simulink model "Capstone_Model"  (R2022b)
settings: Solver=VariableStepAuto  StartTime=0.0  StopTime=10.0  RelTol=1e-3
libraries: sh_lib x6, fl_lib x5, nesl_utility x2, simulink x1
settings Model: Creator=jrodd  LastModifiedBy=jrodd

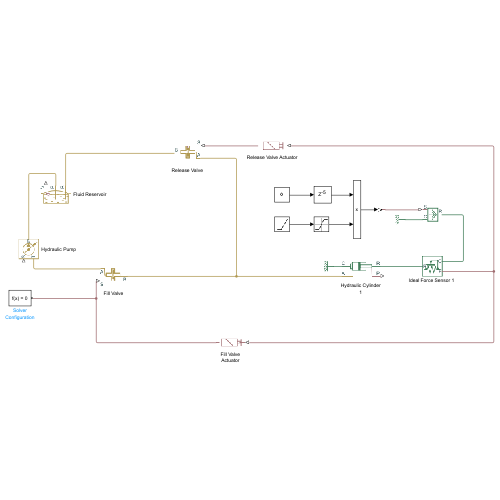
[thumbnail: Simulink's stored preview of the top-level diagram]
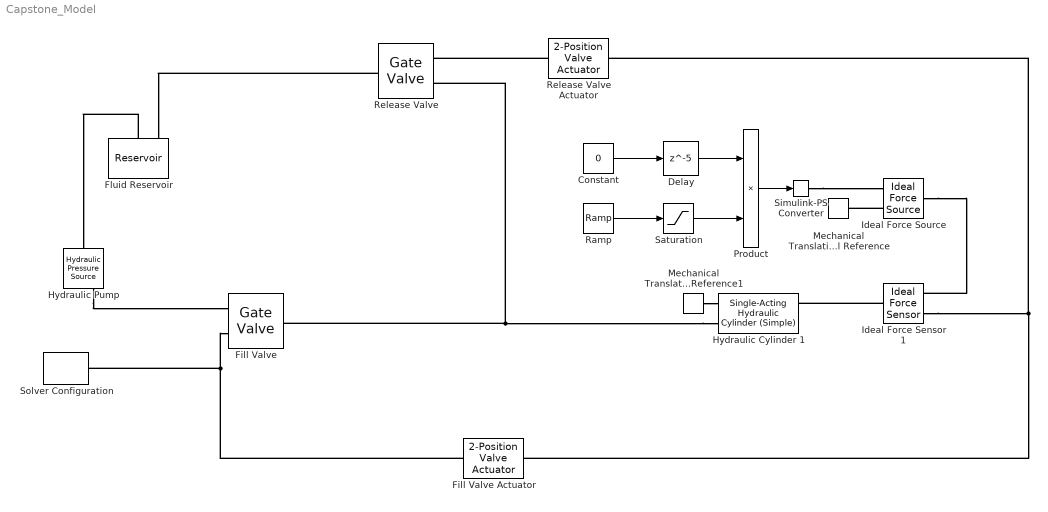
== system Capstone_Model ==
  Constant : Constant  Value=0
  Delay : Delay  DelayLength=5
  Fill Valve : sh_lib/Valves/Flow Control Valves/Gate Valve  d_gate=0.01 m  x_0=0 m  C_d=0.65  A_leak=1e-12 m^2  lam_spec=1  B_lam=0.999  Re_cr=10
      settings: InternalSimscapePortConfiguration="{\"Bottom\":[],\"Left\":[{\"id\":\"S\",\"label\":\"S\",\"type\":\"input\"},{\"id\":\"A\",\"label\":\"A\",\"type\":\"foundation.hydraulic.hydraulic\"}],\"Right\":[{\"id\":\"B\",\"label\":\"B\",\"type\":\"foundation.hydraulic.hydraulic\"}],\"Top\":[]}"
  Fill Valve Actuator : sh_lib/Valves/Valve Actuators/2-Position Valve Actuator  stroke=0.01 m  t_on=0.1 s  t_off=0.1 s  act_signal=1  init_position=0  act_orientation=1
      settings: InternalSimscapePortConfiguration="{\"Bottom\":[],\"Left\":[{\"id\":\"C\",\"label\":\"\",\"type\":\"input\"}],\"Right\":[{\"id\":\"P\",\"label\":\"\",\"type\":\"output\"}],\"Top\":[]}"
  Fluid Reservoir : sh_lib/Hydraulic Utilities/Reservoir  press=0 Pa  init_volume=0.02 m^3  ret_diam=0.02 m  loss_coeff=1
      settings: InternalSimscapePortConfiguration="{\"Bottom\":[],\"Left\":[{\"id\":\"V\",\"label\":\"V\",\"type\":\"output\"},{\"id\":\"P\",\"label\":\"P\",\"type\":\"foundation.hydraulic.hydraulic\"},{\"id\":\"R\",\"label\":\"R\",\"type\":\"foundation.hydraulic.hydraulic\"}],\"Right\":[],\"Top\":[]}"
  Hydraulic Cylinder 1 : sh_lib/Hydraulic Cylinders/Single-Acting Hydraulic Cylinder (Simple)  area=5e-4 m^2  stroke=0.1 m  init_pos=0 m  penetr_coeff=1e12 N*s/m^2  or=1
      settings: InternalSimscapePortConfiguration="{\"Bottom\":[],\"Left\":[{\"id\":\"C\",\"label\":\"C\",\"type\":\"foundation.mechanical.translational.translational\"},{\"id\":\"A\",\"label\":\"A\",\"type\":\"foundation.hydraulic.hydraulic\"}],\"Right\":[{\"id\":\"R\",\"label\":\"R\",\"type\":\"foundation.mechanical.translational.translational\"},{\"id\":\"P\",\"label\":\"P\",\"type\":\"output\"}],\"Top\":[]}"
  Hydraulic Pump : fl_lib/Hydraulic/Hydraulic Sources/Hydraulic Pressure Source
      settings: InternalSimscapePortConfiguration="{\"Bottom\":[],\"Left\":[{\"id\":\"P\",\"label\":\"P\",\"type\":\"foundation.hydraulic.hydraulic\"}],\"Right\":[{\"id\":\"S\",\"label\":\"S\",\"type\":\"input\"},{\"id\":\"T\",\"label\":\"T\",\"type\":\"foundation.hydraulic.hydraulic\"}],\"Top\":[]}"
  "Ideal Force Sensor 1 " : fl_lib/Mechanical/Mechanical Sensors/Ideal Force Sensor
  Ideal Force Source : fl_lib/Mechanical/Mechanical Sources/Ideal Force Source
  Mechanical Translational Reference : fl_lib/Mechanical/Translational Elements/Mechanical Translational Reference
  Mechanical Translational Reference1 : fl_lib/Mechanical/Translational Elements/Mechanical Translational Reference
  Product : Product
  Ramp : simulink/Sources/Ramp  slope=1  start=1  InitialOutput=0
  Release Valve : sh_lib/Valves/Flow Control Valves/Gate Valve  d_gate=0.01 m  x_0=0 m  C_d=0.65  A_leak=1e-12 m^2  lam_spec=1  B_lam=0.999  Re_cr=10
      settings: InternalSimscapePortConfiguration="{\"Bottom\":[],\"Left\":[{\"id\":\"S\",\"label\":\"S\",\"type\":\"input\"},{\"id\":\"A\",\"label\":\"A\",\"type\":\"foundation.hydraulic.hydraulic\"}],\"Right\":[{\"id\":\"B\",\"label\":\"B\",\"type\":\"foundation.hydraulic.hydraulic\"}],\"Top\":[]}"
  Release Valve Actuator : sh_lib/Valves/Valve Actuators/2-Position Valve Actuator  stroke=0.01 m  t_on=0.1 s  t_off=0.1 s  act_signal=1  init_position=1  act_orientation=1
      settings: InternalSimscapePortConfiguration="{\"Bottom\":[],\"Left\":[{\"id\":\"C\",\"label\":\"\",\"type\":\"input\"}],\"Right\":[{\"id\":\"P\",\"label\":\"\",\"type\":\"output\"}],\"Top\":[]}"
  Saturation : Saturate  UpperLimit=2  LowerLimit=0
  Simulink-PS Converter : nesl_utility/Simulink-PS Converter  PhysicalDomain=network_engine_domain  SubClassName=ps_input  LeftPortType=input  RightPortType=output  PseudoPeriodic=off  Frequencies=[]  NoiseDistribution=none  NoiseParameters=[]  Unit=1  AffineConversion=off  FilteringAndDerivatives=provide  SimscapeFilterOrder=1  InputFilterTimeConstant=0.001  UdotUserProvided=0
  Solver Configuration : nesl_utility/Solver Configuration  PhysicalDomain=network_engine_domain  SubClassName=solver  LeftPortType=input  RightPortType=generic  Tones=[]  Harmonics=[]  SimulateNoise=off  Profile=off  UseLocalSampling=off  EnableSwitchedLinearOptims=on  FrequencyDomain=off  UseCCode=off  RelTol=0.001  AbsTol=0.001  MinStep=1e-09  ToWorkspace=off  RevertToSquareIcSolve=off  NumHomotopyIterations=100  PhasorMode=off  PhasorModeNumHarmonics=1  ConsistencySolver=NEWTON_XTOL_AFTER_FTOL  IndexReductionMethod=DerivativeReplacement  DoDC=off  ResidualTolerance=1e-09  ConsistencyTolSource=GLOBAL  ConsistencyAbsTol=0.001  ConsistencyRelTol=0.001  ConsistencyTolFactor=0.001  UseLocalSolver=off  LocalSolverChoice=NE_BACKWARD_EULER_ADVANCER  ResolveIndetEquations=on  FunctionEvalNumThread=1  LocalSolverSampleTime=0.001  DoFixedCost=off  MaxNonlinIter=3  MaxModeIter=2  ComputeImpulses=off  ImpulseIterations=2  LinearAlgebra=auto  LinearAlgebraNumThread=0  EquationFormulation=NE_TIME_EF  DelaysMemoryBudget=1024  AutomaticFiltering=on  FilteringTimeConstant=0.001  PartitionStorageMethod=AS_NEEDED  PartitionMemoryBudget=1024  PartitionMethod=ROBUST
  wires:
  Ramp/1 -> Saturation/1
  Saturation/1 -> Product/2
  Product/1 -> Simulink-PS Converter/1
  Constant/1 -> Delay/1
  Delay/1 -> Product/1
  connections:
  Hydraulic Cylinder 1/LConn2 -- Fill Valve/RConn1 -- Release Valve/LConn2
  Fill Valve Actuator/RConn1 -- Solver Configuration/RConn1 -- Fill Valve/LConn1
  Hydraulic Pump/RConn2 -- Fill Valve/LConn2
  Release Valve Actuator/RConn1 -- Release Valve/LConn1
  Fluid Reservoir/LConn2 -- Hydraulic Pump/LConn1
  Release Valve/RConn1 -- Fluid Reservoir/LConn3
  "Ideal Force Sensor 1 "/LConn1 -- Hydraulic Cylinder 1/RConn1
  "Ideal Force Sensor 1 "/RConn2 -- Release Valve Actuator/LConn1 -- Fill Valve Actuator/LConn1
  Ideal Force Source/LConn1 -- "Ideal Force Sensor 1 "/RConn1
  Simulink-PS Converter/RConn1 -- Ideal Force Source/RConn1
  Ideal Force Source/RConn2 -- Mechanical Translational Reference/LConn1
  Mechanical Translational Reference1/LConn1 -- Hydraulic Cylinder 1/LConn1
